simulink model "TEST_SensorSource_FromWorkspace"  (R2020b)
settings: Solver=ode1  StartTime=tspan(1)  StopTime=tspan(2)  FixedStep=1/sensorFs.imuUpdateFs  RelTol=1e-3
values from neighbouring files (symbols this model uses):
  mag1 = double([Sensors.mag1.mag_x, Sensors.mag1.mag_y, Sensors.mag1.mag_z])    [navi_marg22.m]    (also in navi_marg24.m; navi_mvo17.m)
  mag2 = double([Sensors.mag2.mag_x, Sensors.mag2.mag_y, Sensors.mag2.mag_z])    [navi_marg22.m]    (also in navi_marg24.m; navi_mvo17.m)
  time = naviRes.time    [Plot_NaviMARG.m]    (also in UAVPlotLib.m = sensors.(sensorName).time; myplot_navfilter.m = sensors.Algo.time_algo; myplot_sensor_filter_compare.m = sensors.IMU.time_imu; postplot_marg_flightdata.m = sensors.Algo.time_algo)
undefined symbols (not defined in the file or in its folder): airspeed1, airspeed2, airspeed3, baro1, IMU1, IMU1_Control, IMU2, IMU3, IN_SENSOR_SIM, laserDown1, laserDown2, radar1, radarLongDown1, radarLongForward1, ublox1, um482
settings Model: PauseTimes=266.88  Creator=sl  LastModifiedBy=sl
settings SolverCC: AutoInsertRateTranBlk=on
settings OptimizationCC: DefaultParameterBehavior=Inlined  EnhancedBackFolding=on  PassReuseOutputArgsAs=Individual arguments  ZeroExternalMemoryAtStartup=off  ZeroInternalMemoryAtStartup=off  MaxStackSize=64  OptimizeBlockOrder=speed  DifferentSizesBufferReuse=on  OptimizationCustomize=off  EfficientTunableParamExpr=on
settings DebuggingCC: MultiTaskCondExecSysMsg=none  ParameterPrecisionLossMsg=none  ParameterTunabilityLossMsg=error  UnconnectedInputMsg=none  UnconnectedOutputMsg=none  UnconnectedLineMsg=none  BusObjectLabelMismatch=error
settings HardwareCC: ProdBitPerPointer=32  ProdBitPerSizeT=32  ProdBitPerPtrDiffT=32  ProdLargestAtomicInteger=Long  ProdLargestAtomicFloat=Double  ProdWordSize=32  ProdHWDeviceType=ARM Compatible->ARM Cortex
settings ModelReferenceCC: EnableParallelModelReferenceBuilds=on  ParallelModelReferenceMATLABWorkerInit=Load Top Model
settings SFSimCC: MATLABDynamicMemAlloc=off
settings RTWCC: Description=Embedded Coder  SystemTargetFile=ert.tlc  TemplateMakefile=ert_default_tmf  GenerateReport=on  Toolchain=GNU Tools for ARM Embedded Processors  IncludeHyperlinkInReport=on  LaunchReport=on  GenerateTraceInfo=on  GenerateTraceReport=on  GenerateTraceReportSl=on  GenerateTraceReportSf=on  GenerateTraceReportEml=on
settings CodeAppCC: ForceParamTrailComments=on  IgnoreCustomStorageClasses=off  OperatorAnnotations=on  SimulinkDataObjDesc=on  SFDataObjDesc=on  InsertBlockDesc=on
settings ERTTargetCC: InlinedParameterPlacement=NonHierarchical  ERTCustomFileTemplate=example_file_process.tlc

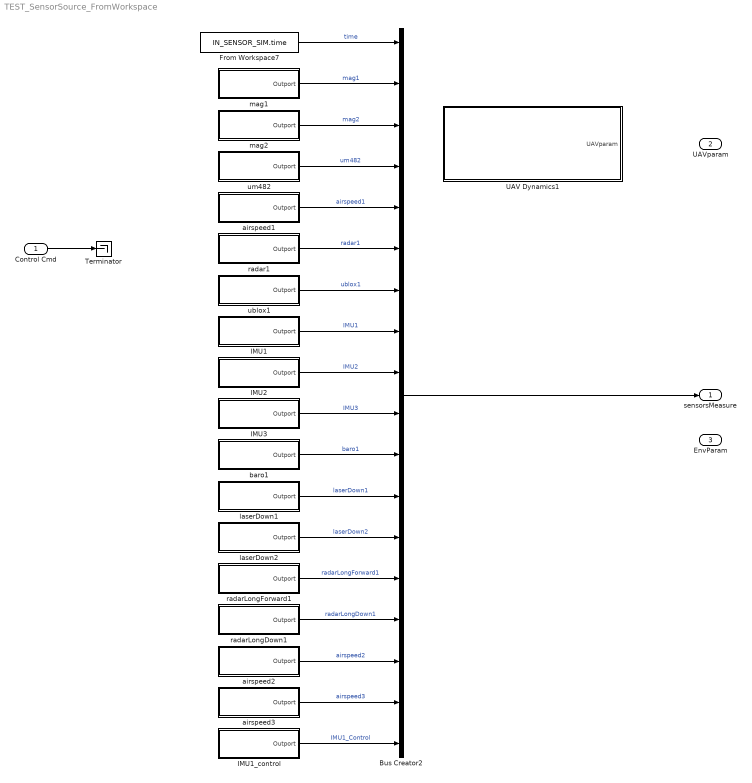
== system TEST_SensorSource_FromWorkspace ==
  Control Cmd : Inport  OutDataTypeStr=Bus: BUS_CONTROL_ACTUATOR
  Bus Creator2 : BusCreator  Inputs=time,mag1,mag2,um482,airspeed1,radar1,ublox1,IMU1,IMU2,IMU3,baro1,laserDown1,laserDown2,radarLongForward1,radarLongDown1,airspeed2,airspeed3,IMU1_Control  OutDataTypeStr=Bus: BUS_SENSOR
  From Workspace7 : FromWorkspace  VariableName=IN_SENSOR_SIM.time  OutputAfterFinalValue=Holding final value
  IMU1 : Subsystem  mask{data=IN_SENSOR_SIM.IMU1}
      mask prompts: data "IMU数据结构体"
  IMU1_control : Subsystem  mask{data=IN_SENSOR_SIM.IMU1_Control}
      mask prompts: data "IMU数据结构体"
  IMU2 : Subsystem  mask{data=IN_SENSOR_SIM.IMU2}
      mask prompts: data "IMU数据结构体"
  IMU3 : Subsystem  mask{data=IN_SENSOR_SIM.IMU3}
      mask prompts: data "IMU数据结构体"
  Terminator : Terminator
  UAV Dynamics1 : Subsystem
  airspeed1 : Subsystem  mask{data=IN_SENSOR_SIM.airspeed1}
      mask prompts: data "airspeed数据结构体"
  airspeed2 : Subsystem  mask{data=IN_SENSOR_SIM.airspeed2}
      mask prompts: data "airspeed数据结构体"
  airspeed3 : Subsystem  mask{data=IN_SENSOR_SIM.airspeed3}
      mask prompts: data "airspeed数据结构体"
  baro1 : Subsystem  mask{data=IN_SENSOR_SIM.baro1}
      mask prompts: data "baro数据结构体"
  laserDown1 : Subsystem  mask{data=IN_SENSOR_SIM.laserDown2}
      mask prompts: data "baro数据结构体"
  laserDown2 : Subsystem  mask{data=IN_SENSOR_SIM.laserDown2}
      mask prompts: data "baro数据结构体"
  mag1 : Subsystem  mask{data=IN_SENSOR_SIM.mag1}
      mask prompts: data "mag数据结构体"
  mag2 : Subsystem  mask{data=IN_SENSOR_SIM.mag2}
      mask prompts: data "mag数据结构体"
  radar1 : Subsystem  mask{data=IN_SENSOR_SIM.radar1}
      mask prompts: data "radar数据结构体"
  radarLongDown1 : Subsystem  mask{data=IN_SENSOR_SIM.radarLongDown1}
      mask prompts: data "baro数据结构体"
  radarLongForward1 : Subsystem  mask{data=IN_SENSOR_SIM.radarLongForward1}
      mask prompts: data "baro数据结构体"
  ublox1 : Subsystem  mask{data=IN_SENSOR_SIM.ublox1}
      mask prompts: data "ublox数据结构体"
  um482 : Subsystem  mask{data=IN_SENSOR_SIM.um482}
      mask prompts: data "um482数据结构体"
  sensorsMeasure : Outport  OutDataTypeStr=Bus: BUS_SENSOR
  UAVparam : Outport  Port=2  OutDataTypeStr=Bus: BUS_UAVDYN_FlightParam
  EnvParam : Outport  Port=3  OutDataTypeStr=Bus: BUS_UAVDYN_Env  LockScale=on
  wires:
  um482/1(Outport) -> Bus Creator2/4  "um482"
  Control Cmd/1 -> Terminator/1
  radarLongForward1/1(Outport) -> Bus Creator2/14  "radarLongForward1"
  radar1/1(Outport) -> Bus Creator2/6  "radar1"
  mag2/1(Outport) -> Bus Creator2/3  "mag2"
  airspeed2/1(Outport) -> Bus Creator2/16  "airspeed2"
  IMU2/1(Outport) -> Bus Creator2/9  "IMU2"
  airspeed1/1(Outport) -> Bus Creator2/5  "airspeed1"
  radarLongDown1/1(Outport) -> Bus Creator2/15  "radarLongDown1"
  From Workspace7/1 -> Bus Creator2/1  "time"
  mag1/1(Outport) -> Bus Creator2/2  "mag1"
  IMU1/1(Outport) -> Bus Creator2/8  "IMU1"
  airspeed3/1(Outport) -> Bus Creator2/17  "airspeed3"
  Bus Creator2/1 -> sensorsMeasure/1
  IMU1_control/1(Outport) -> Bus Creator2/18  "IMU1_Control"
  laserDown1/1(Outport) -> Bus Creator2/12  "laserDown1"
  baro1/1(Outport) -> Bus Creator2/11  "baro1"
  ublox1/1(Outport) -> Bus Creator2/7  "ublox1"
  laserDown2/1(Outport) -> Bus Creator2/13  "laserDown2"
  IMU3/1(Outport) -> Bus Creator2/10  "IMU3"

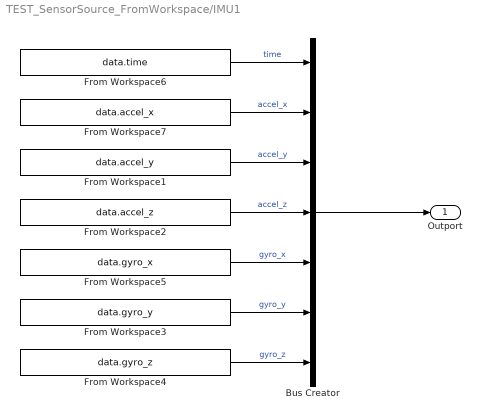
== system TEST_SensorSource_FromWorkspace/IMU1 ==
  Bus Creator : BusCreator  Inputs=7
  From Workspace1 : FromWorkspace  VariableName=data.accel_y  OutputAfterFinalValue=Holding final value
  From Workspace2 : FromWorkspace  VariableName=data.accel_z  OutputAfterFinalValue=Holding final value
  From Workspace3 : FromWorkspace  VariableName=data.gyro_y  OutputAfterFinalValue=Holding final value
  From Workspace4 : FromWorkspace  VariableName=data.gyro_z  OutputAfterFinalValue=Holding final value
  From Workspace5 : FromWorkspace  VariableName=data.gyro_x  OutputAfterFinalValue=Holding final value
  From Workspace6 : FromWorkspace  VariableName=data.time  OutputAfterFinalValue=Holding final value
  From Workspace7 : FromWorkspace  VariableName=data.accel_x  OutputAfterFinalValue=Holding final value
  Outport : Outport
  wires:
  From Workspace1/1 -> Bus Creator/3  "accel_y"
  From Workspace4/1 -> Bus Creator/7  "gyro_z"
  Bus Creator/1 -> Outport/1
  From Workspace2/1 -> Bus Creator/4  "accel_z"
  From Workspace5/1 -> Bus Creator/5  "gyro_x"
  From Workspace7/1 -> Bus Creator/2  "accel_x"
  From Workspace6/1 -> Bus Creator/1  "time"
  From Workspace3/1 -> Bus Creator/6  "gyro_y"

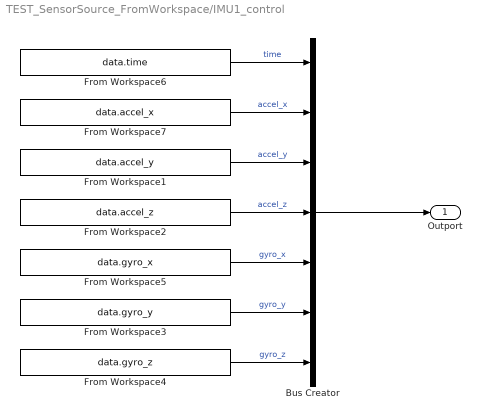
== system TEST_SensorSource_FromWorkspace/IMU1_control ==
  Bus Creator : BusCreator  Inputs=7
  From Workspace1 : FromWorkspace  VariableName=data.accel_y  OutputAfterFinalValue=Holding final value
  From Workspace2 : FromWorkspace  VariableName=data.accel_z  OutputAfterFinalValue=Holding final value
  From Workspace3 : FromWorkspace  VariableName=data.gyro_y  OutputAfterFinalValue=Holding final value
  From Workspace4 : FromWorkspace  VariableName=data.gyro_z  OutputAfterFinalValue=Holding final value
  From Workspace5 : FromWorkspace  VariableName=data.gyro_x  OutputAfterFinalValue=Holding final value
  From Workspace6 : FromWorkspace  VariableName=data.time  OutputAfterFinalValue=Holding final value
  From Workspace7 : FromWorkspace  VariableName=data.accel_x  OutputAfterFinalValue=Holding final value
  Outport : Outport
  wires:
  From Workspace3/1 -> Bus Creator/6  "gyro_y"
  From Workspace6/1 -> Bus Creator/1  "time"
  From Workspace7/1 -> Bus Creator/2  "accel_x"
  From Workspace5/1 -> Bus Creator/5  "gyro_x"
  From Workspace2/1 -> Bus Creator/4  "accel_z"
  Bus Creator/1 -> Outport/1
  From Workspace4/1 -> Bus Creator/7  "gyro_z"
  From Workspace1/1 -> Bus Creator/3  "accel_y"

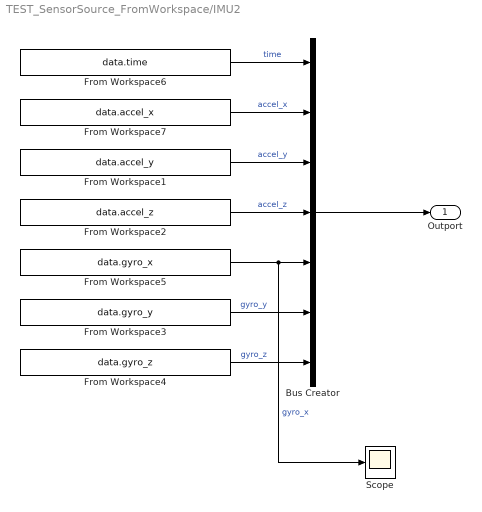
== system TEST_SensorSource_FromWorkspace/IMU2 ==
  Bus Creator : BusCreator  Inputs=7
  From Workspace1 : FromWorkspace  VariableName=data.accel_y  OutputAfterFinalValue=Holding final value
  From Workspace2 : FromWorkspace  VariableName=data.accel_z  OutputAfterFinalValue=Holding final value
  From Workspace3 : FromWorkspace  VariableName=data.gyro_y  OutputAfterFinalValue=Holding final value
  From Workspace4 : FromWorkspace  VariableName=data.gyro_z  OutputAfterFinalValue=Holding final value
  From Workspace5 : FromWorkspace  VariableName=data.gyro_x  OutputAfterFinalValue=Holding final value
  From Workspace6 : FromWorkspace  VariableName=data.time  OutputAfterFinalValue=Holding final value
  From Workspace7 : FromWorkspace  VariableName=data.accel_x  OutputAfterFinalValue=Holding final value
  Scope : Scope
  Outport : Outport
  wires:
  From Workspace3/1 -> Bus Creator/6  "gyro_y"
  From Workspace6/1 -> Bus Creator/1  "time"
  From Workspace7/1 -> Bus Creator/2  "accel_x"
  From Workspace5/1 -> Scope/1, Bus Creator/5  "gyro_x"
  From Workspace2/1 -> Bus Creator/4  "accel_z"
  Bus Creator/1 -> Outport/1
  From Workspace4/1 -> Bus Creator/7  "gyro_z"
  From Workspace1/1 -> Bus Creator/3  "accel_y"

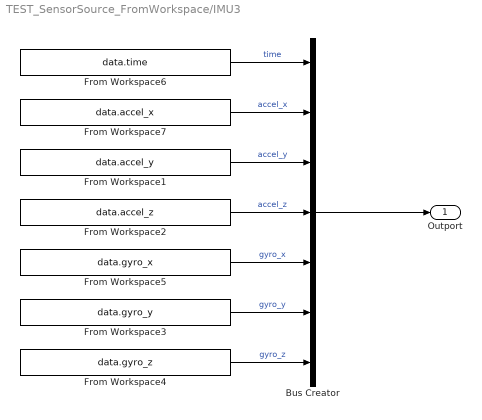
== system TEST_SensorSource_FromWorkspace/IMU3 ==
  Bus Creator : BusCreator  Inputs=7
  From Workspace1 : FromWorkspace  VariableName=data.accel_y  OutputAfterFinalValue=Holding final value
  From Workspace2 : FromWorkspace  VariableName=data.accel_z  OutputAfterFinalValue=Holding final value
  From Workspace3 : FromWorkspace  VariableName=data.gyro_y  OutputAfterFinalValue=Holding final value
  From Workspace4 : FromWorkspace  VariableName=data.gyro_z  OutputAfterFinalValue=Holding final value
  From Workspace5 : FromWorkspace  VariableName=data.gyro_x  OutputAfterFinalValue=Holding final value
  From Workspace6 : FromWorkspace  VariableName=data.time  OutputAfterFinalValue=Holding final value
  From Workspace7 : FromWorkspace  VariableName=data.accel_x  OutputAfterFinalValue=Holding final value
  Outport : Outport
  wires:
  From Workspace1/1 -> Bus Creator/3  "accel_y"
  From Workspace4/1 -> Bus Creator/7  "gyro_z"
  Bus Creator/1 -> Outport/1
  From Workspace2/1 -> Bus Creator/4  "accel_z"
  From Workspace5/1 -> Bus Creator/5  "gyro_x"
  From Workspace7/1 -> Bus Creator/2  "accel_x"
  From Workspace6/1 -> Bus Creator/1  "time"
  From Workspace3/1 -> Bus Creator/6  "gyro_y"

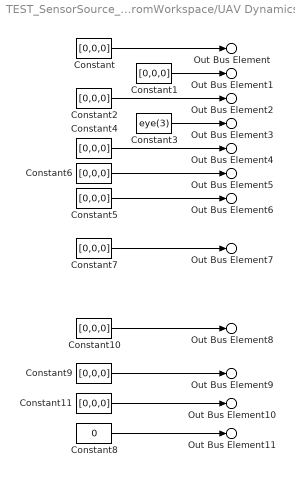
== system TEST_SensorSource_FromWorkspace/UAV Dynamics1 ==
  Constant{,1..2,4..7,9..11} (10 alike) : Constant  Value=[0,0,0]
  Constant3 : Constant  Value=eye(3)
  Constant8 : Constant  Value=0
  Out Bus Element : Outport  PortName=UAVparam  Element=vel_NED
  Out Bus Element1 : Outport  PortName=UAVparam  Element=pos_NED
  Out Bus Element2 : Outport  PortName=UAVparam  Element=euler_yaw_pitch_roll
  Out Bus Element3 : Outport  PortName=UAVparam  Element=DCMbe
  Out Bus Element4 : Outport  PortName=UAVparam  Element=vel_Body
  Out Bus Element5 : Outport  PortName=UAVparam  Element=w_Body
  Out Bus Element6 : Outport  PortName=UAVparam  Element=dw_Body
  Out Bus Element7 : Outport  PortName=UAVparam  Element=LLA
  Out Bus Element8 : Outport  PortName=UAVparam  Element=specificForce_Body
  Out Bus Element9 : Outport  PortName=UAVparam  Element=mag_Body
  Out Bus Element10 : Outport  PortName=UAVparam  Element=mag_NED
  Out Bus Element11 : Outport  PortName=UAVparam  Element=magDec_deg
  wires:
  Constant/1 -> Out Bus Element/1
  Constant1/1 -> Out Bus Element1/1
  Constant2/1 -> Out Bus Element2/1
  Constant3/1 -> Out Bus Element3/1
  Constant4/1 -> Out Bus Element4/1
  Constant6/1 -> Out Bus Element5/1
  Constant5/1 -> Out Bus Element6/1
  Constant7/1 -> Out Bus Element7/1
  Constant10/1 -> Out Bus Element8/1
  Constant9/1 -> Out Bus Element9/1
  Constant11/1 -> Out Bus Element10/1
  Constant8/1 -> Out Bus Element11/1

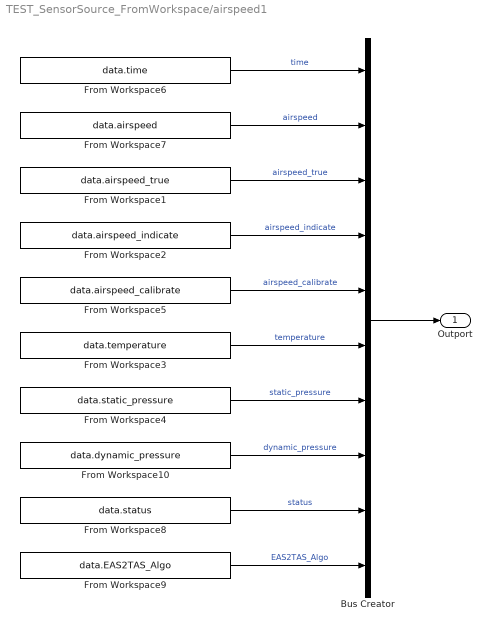
== system TEST_SensorSource_FromWorkspace/airspeed1 ==
  Bus Creator : BusCreator  Inputs=10
  From Workspace1 : FromWorkspace  VariableName=data.airspeed_true  OutputAfterFinalValue=Holding final value
  From Workspace10 : FromWorkspace  VariableName=data.dynamic_pressure  OutputAfterFinalValue=Holding final value
  From Workspace2 : FromWorkspace  VariableName=data.airspeed_indicate  OutputAfterFinalValue=Holding final value
  From Workspace3 : FromWorkspace  VariableName=data.temperature  OutputAfterFinalValue=Holding final value
  From Workspace4 : FromWorkspace  VariableName=data.static_pressure  OutputAfterFinalValue=Holding final value
  From Workspace5 : FromWorkspace  VariableName=data.airspeed_calibrate  OutputAfterFinalValue=Holding final value
  From Workspace6 : FromWorkspace  VariableName=data.time  OutputAfterFinalValue=Holding final value
  From Workspace7 : FromWorkspace  VariableName=data.airspeed  OutputAfterFinalValue=Holding final value
  From Workspace8 : FromWorkspace  VariableName=data.status  OutputAfterFinalValue=Holding final value
  From Workspace9 : FromWorkspace  VariableName=data.EAS2TAS_Algo  OutputAfterFinalValue=Holding final value
  Outport : Outport
  wires:
  Bus Creator/1 -> Outport/1
  From Workspace7/1 -> Bus Creator/2  "airspeed"
  From Workspace6/1 -> Bus Creator/1  "time"
  From Workspace1/1 -> Bus Creator/3  "airspeed_true"
  From Workspace2/1 -> Bus Creator/4  "airspeed_indicate"
  From Workspace5/1 -> Bus Creator/5  "airspeed_calibrate"
  From Workspace3/1 -> Bus Creator/6  "temperature"
  From Workspace4/1 -> Bus Creator/7  "static_pressure"
  From Workspace10/1 -> Bus Creator/8  "dynamic_pressure"
  From Workspace8/1 -> Bus Creator/9  "status"
  From Workspace9/1 -> Bus Creator/10  "EAS2TAS_Algo"

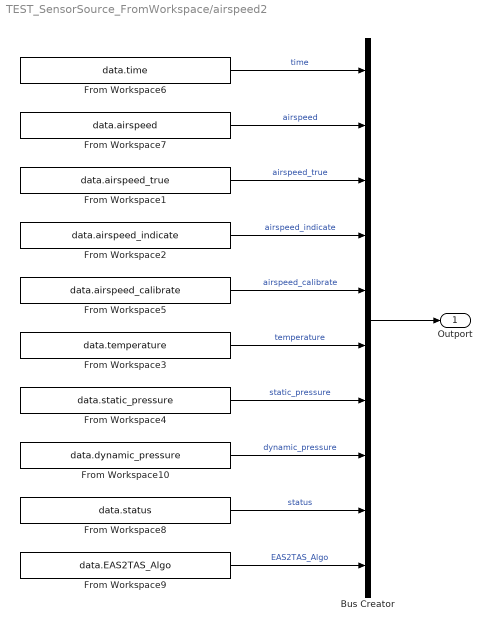
== system TEST_SensorSource_FromWorkspace/airspeed2 ==
  Bus Creator : BusCreator  Inputs=10
  From Workspace1 : FromWorkspace  VariableName=data.airspeed_true  OutputAfterFinalValue=Holding final value
  From Workspace10 : FromWorkspace  VariableName=data.dynamic_pressure  OutputAfterFinalValue=Holding final value
  From Workspace2 : FromWorkspace  VariableName=data.airspeed_indicate  OutputAfterFinalValue=Holding final value
  From Workspace3 : FromWorkspace  VariableName=data.temperature  OutputAfterFinalValue=Holding final value
  From Workspace4 : FromWorkspace  VariableName=data.static_pressure  OutputAfterFinalValue=Holding final value
  From Workspace5 : FromWorkspace  VariableName=data.airspeed_calibrate  OutputAfterFinalValue=Holding final value
  From Workspace6 : FromWorkspace  VariableName=data.time  OutputAfterFinalValue=Holding final value
  From Workspace7 : FromWorkspace  VariableName=data.airspeed  OutputAfterFinalValue=Holding final value
  From Workspace8 : FromWorkspace  VariableName=data.status  OutputAfterFinalValue=Holding final value
  From Workspace9 : FromWorkspace  VariableName=data.EAS2TAS_Algo  OutputAfterFinalValue=Holding final value
  Outport : Outport
  wires:
  From Workspace8/1 -> Bus Creator/9  "status"
  From Workspace10/1 -> Bus Creator/8  "dynamic_pressure"
  From Workspace6/1 -> Bus Creator/1  "time"
  From Workspace2/1 -> Bus Creator/4  "airspeed_indicate"
  From Workspace5/1 -> Bus Creator/5  "airspeed_calibrate"
  Bus Creator/1 -> Outport/1
  From Workspace7/1 -> Bus Creator/2  "airspeed"
  From Workspace1/1 -> Bus Creator/3  "airspeed_true"
  From Workspace4/1 -> Bus Creator/7  "static_pressure"
  From Workspace3/1 -> Bus Creator/6  "temperature"
  From Workspace9/1 -> Bus Creator/10  "EAS2TAS_Algo"

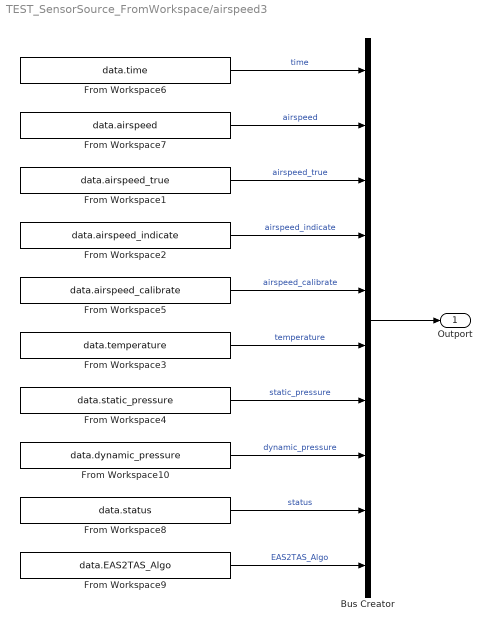
== system TEST_SensorSource_FromWorkspace/airspeed3 ==
  Bus Creator : BusCreator  Inputs=10
  From Workspace1 : FromWorkspace  VariableName=data.airspeed_true  OutputAfterFinalValue=Holding final value
  From Workspace10 : FromWorkspace  VariableName=data.dynamic_pressure  OutputAfterFinalValue=Holding final value
  From Workspace2 : FromWorkspace  VariableName=data.airspeed_indicate  OutputAfterFinalValue=Holding final value
  From Workspace3 : FromWorkspace  VariableName=data.temperature  OutputAfterFinalValue=Holding final value
  From Workspace4 : FromWorkspace  VariableName=data.static_pressure  OutputAfterFinalValue=Holding final value
  From Workspace5 : FromWorkspace  VariableName=data.airspeed_calibrate  OutputAfterFinalValue=Holding final value
  From Workspace6 : FromWorkspace  VariableName=data.time  OutputAfterFinalValue=Holding final value
  From Workspace7 : FromWorkspace  VariableName=data.airspeed  OutputAfterFinalValue=Holding final value
  From Workspace8 : FromWorkspace  VariableName=data.status  OutputAfterFinalValue=Holding final value
  From Workspace9 : FromWorkspace  VariableName=data.EAS2TAS_Algo  OutputAfterFinalValue=Holding final value
  Outport : Outport
  wires:
  From Workspace8/1 -> Bus Creator/9  "status"
  From Workspace10/1 -> Bus Creator/8  "dynamic_pressure"
  From Workspace6/1 -> Bus Creator/1  "time"
  From Workspace2/1 -> Bus Creator/4  "airspeed_indicate"
  From Workspace5/1 -> Bus Creator/5  "airspeed_calibrate"
  Bus Creator/1 -> Outport/1
  From Workspace7/1 -> Bus Creator/2  "airspeed"
  From Workspace1/1 -> Bus Creator/3  "airspeed_true"
  From Workspace4/1 -> Bus Creator/7  "static_pressure"
  From Workspace3/1 -> Bus Creator/6  "temperature"
  From Workspace9/1 -> Bus Creator/10  "EAS2TAS_Algo"

== system TEST_SensorSource_FromWorkspace/baro1 ==
  Bus Creator : BusCreator  Inputs=2
  From Workspace6 : FromWorkspace  VariableName=data.time  OutputAfterFinalValue=Holding final value
  From Workspace7 : FromWorkspace  VariableName=data.alt_baro  OutputAfterFinalValue=Holding final value
  Outport : Outport
  wires:
  From Workspace6/1 -> Bus Creator/1  "time"
  From Workspace7/1 -> Bus Creator/2  "alt_baro"
  Bus Creator/1 -> Outport/1

== system TEST_SensorSource_FromWorkspace/laserDown1 ==
  Bus Creator : BusCreator  Inputs=4
  From Workspace1 : FromWorkspace  VariableName=data.flag  OutputAfterFinalValue=Holding final value
  From Workspace2 : FromWorkspace  VariableName=data.strength  OutputAfterFinalValue=Holding final value
  From Workspace6 : FromWorkspace  VariableName=data.time  OutputAfterFinalValue=Holding final value
  From Workspace7 : FromWorkspace  VariableName=data.range  OutputAfterFinalValue=Holding final value
  Outport : Outport
  wires:
  Bus Creator/1 -> Outport/1
  From Workspace7/1 -> Bus Creator/2  "range"
  From Workspace6/1 -> Bus Creator/1  "time"
  From Workspace1/1 -> Bus Creator/3  "flag"
  From Workspace2/1 -> Bus Creator/4  "strength"

== system TEST_SensorSource_FromWorkspace/laserDown2 ==
  Bus Creator : BusCreator  Inputs=4
  From Workspace1 : FromWorkspace  VariableName=data.flag  OutputAfterFinalValue=Holding final value
  From Workspace2 : FromWorkspace  VariableName=data.strength  OutputAfterFinalValue=Holding final value
  From Workspace6 : FromWorkspace  VariableName=data.time  OutputAfterFinalValue=Holding final value
  From Workspace7 : FromWorkspace  VariableName=data.range  OutputAfterFinalValue=Holding final value
  Outport : Outport
  wires:
  From Workspace2/1 -> Bus Creator/4  "strength"
  From Workspace1/1 -> Bus Creator/3  "flag"
  From Workspace6/1 -> Bus Creator/1  "time"
  From Workspace7/1 -> Bus Creator/2  "range"
  Bus Creator/1 -> Outport/1

== system TEST_SensorSource_FromWorkspace/mag1 ==
  Bus Creator : BusCreator  Inputs=4
  From Workspace6 : FromWorkspace  VariableName=data.time  OutputAfterFinalValue=Holding final value
  mag_x : FromWorkspace  VariableName=data.mag_x  OutputAfterFinalValue=Holding final value
  mag_y : FromWorkspace  VariableName=data.mag_y  OutputAfterFinalValue=Holding final value
  mag_z : FromWorkspace  VariableName=data.mag_z  OutputAfterFinalValue=Holding final value
  Outport : Outport
  wires:
  From Workspace6/1 -> Bus Creator/1  "time"
  mag_x/1 -> Bus Creator/2  "mag_x"
  mag_z/1 -> Bus Creator/4  "mag_z"
  Bus Creator/1 -> Outport/1
  mag_y/1 -> Bus Creator/3  "mag_y"

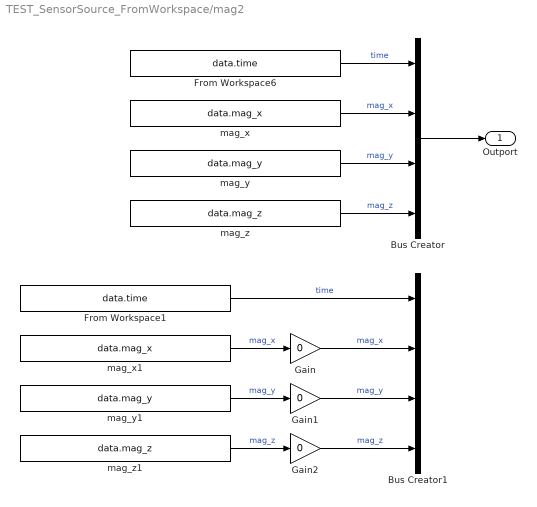
== system TEST_SensorSource_FromWorkspace/mag2 ==
  Bus Creator : BusCreator  Inputs=4
  Bus Creator1 : BusCreator  Inputs=4
  From Workspace1 : FromWorkspace  VariableName=data.time  OutputAfterFinalValue=Holding final value
  From Workspace6 : FromWorkspace  VariableName=data.time  OutputAfterFinalValue=Holding final value
  Gain : Gain  Gain=0
  Gain1 : Gain  Gain=0
  Gain2 : Gain  Gain=0
  mag_x : FromWorkspace  VariableName=data.mag_x  OutputAfterFinalValue=Holding final value
  mag_x1 : FromWorkspace  VariableName=data.mag_x  OutputAfterFinalValue=Holding final value
  mag_y : FromWorkspace  VariableName=data.mag_y  OutputAfterFinalValue=Holding final value
  mag_y1 : FromWorkspace  VariableName=data.mag_y  OutputAfterFinalValue=Holding final value
  mag_z : FromWorkspace  VariableName=data.mag_z  OutputAfterFinalValue=Holding final value
  mag_z1 : FromWorkspace  VariableName=data.mag_z  OutputAfterFinalValue=Holding final value
  Outport : Outport
  wires:
  mag_y/1 -> Bus Creator/3  "mag_y"
  mag_z/1 -> Bus Creator/4  "mag_z"
  mag_x/1 -> Bus Creator/2  "mag_x"
  From Workspace6/1 -> Bus Creator/1  "time"
  From Workspace1/1 -> Bus Creator1/1  "time"
  mag_x1/1 -> Gain/1  "mag_x"
  mag_z1/1 -> Gain2/1  "mag_z"
  mag_y1/1 -> Gain1/1  "mag_y"
  Gain/1 -> Bus Creator1/2  "mag_x"
  Gain1/1 -> Bus Creator1/3  "mag_y"
  Gain2/1 -> Bus Creator1/4  "mag_z"
  Bus Creator/1 -> Outport/1

== system TEST_SensorSource_FromWorkspace/radar1 ==
  Bus Creator : BusCreator  Inputs=4
  From Workspace1 : FromWorkspace  VariableName=data.Flag  OutputAfterFinalValue=Holding final value
  From Workspace2 : FromWorkspace  VariableName=data.Range  Interpolate=off  OutputAfterFinalValue=Holding final value
  From Workspace6 : FromWorkspace  VariableName=data.time  OutputAfterFinalValue=Holding final value
  From Workspace7 : FromWorkspace  VariableName=data.SNR  OutputAfterFinalValue=Holding final value
  Outport : Outport
  wires:
  From Workspace6/1 -> Bus Creator/1  "time"
  From Workspace7/1 -> Bus Creator/2  "SNR"
  From Workspace2/1 -> Bus Creator/4  "Range"
  Bus Creator/1 -> Outport/1
  From Workspace1/1 -> Bus Creator/3  "Flag"

== system TEST_SensorSource_FromWorkspace/radarLongDown1 ==
  Bus Creator : BusCreator  Inputs=4
  From Workspace1 : FromWorkspace  VariableName=data.flag  OutputAfterFinalValue=Holding final value
  From Workspace2 : FromWorkspace  VariableName=data.strength  OutputAfterFinalValue=Holding final value
  From Workspace6 : FromWorkspace  VariableName=data.time  OutputAfterFinalValue=Holding final value
  From Workspace7 : FromWorkspace  VariableName=data.range  OutputAfterFinalValue=Holding final value
  Outport : Outport
  wires:
  Bus Creator/1 -> Outport/1
  From Workspace7/1 -> Bus Creator/2  "range"
  From Workspace6/1 -> Bus Creator/1  "time"
  From Workspace1/1 -> Bus Creator/3  "flag"
  From Workspace2/1 -> Bus Creator/4  "strength"

== system TEST_SensorSource_FromWorkspace/radarLongForward1 ==
  Bus Creator : BusCreator  Inputs=4
  From Workspace1 : FromWorkspace  VariableName=data.flag  OutputAfterFinalValue=Holding final value
  From Workspace2 : FromWorkspace  VariableName=data.strength  OutputAfterFinalValue=Holding final value
  From Workspace6 : FromWorkspace  VariableName=data.time  OutputAfterFinalValue=Holding final value
  From Workspace7 : FromWorkspace  VariableName=data.range  OutputAfterFinalValue=Holding final value
  Outport : Outport
  wires:
  From Workspace2/1 -> Bus Creator/4  "strength"
  From Workspace1/1 -> Bus Creator/3  "flag"
  From Workspace6/1 -> Bus Creator/1  "time"
  From Workspace7/1 -> Bus Creator/2  "range"
  Bus Creator/1 -> Outport/1

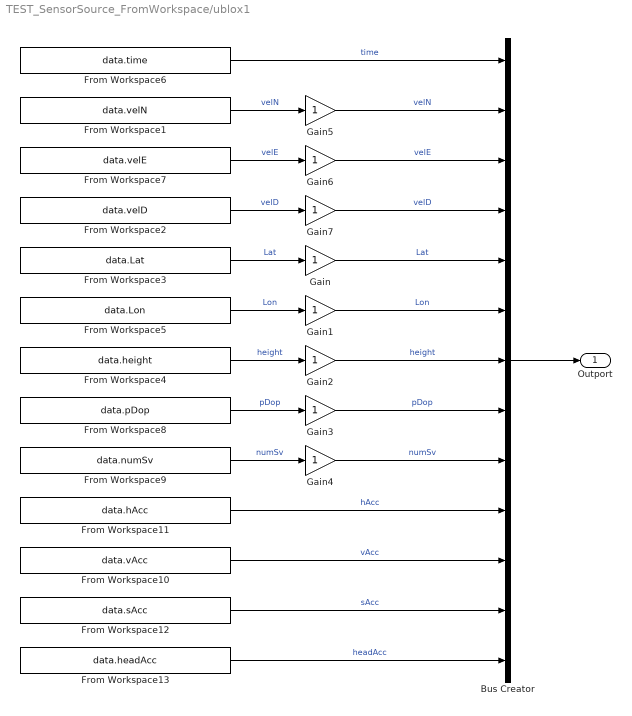
== system TEST_SensorSource_FromWorkspace/ublox1 ==
  Bus Creator : BusCreator  Inputs=13
  From Workspace1 : FromWorkspace  VariableName=data.velN  OutputAfterFinalValue=Holding final value
  From Workspace10 : FromWorkspace  VariableName=data.vAcc  OutputAfterFinalValue=Holding final value
  From Workspace11 : FromWorkspace  VariableName=data.hAcc  OutputAfterFinalValue=Holding final value
  From Workspace12 : FromWorkspace  VariableName=data.sAcc  OutputAfterFinalValue=Holding final value
  From Workspace13 : FromWorkspace  VariableName=data.headAcc  OutputAfterFinalValue=Holding final value
  From Workspace2 : FromWorkspace  VariableName=data.velD  OutputAfterFinalValue=Holding final value
  From Workspace3 : FromWorkspace  VariableName=data.Lat  OutputAfterFinalValue=Holding final value
  From Workspace4 : FromWorkspace  VariableName=data.height  OutputAfterFinalValue=Holding final value
  From Workspace5 : FromWorkspace  VariableName=data.Lon  OutputAfterFinalValue=Holding final value
  From Workspace6 : FromWorkspace  VariableName=data.time  OutputAfterFinalValue=Holding final value
  From Workspace7 : FromWorkspace  VariableName=data.velE  OutputAfterFinalValue=Holding final value
  From Workspace8 : FromWorkspace  VariableName=data.pDop  OutputAfterFinalValue=Holding final value
  From Workspace9 : FromWorkspace  VariableName=data.numSv  OutputAfterFinalValue=Holding final value
  Gain{,1..7} (8 alike) : Gain
  Outport : Outport
  wires:
  From Workspace9/1 -> Gain4/1  "numSv"
  From Workspace8/1 -> Gain3/1  "pDop"
  From Workspace4/1 -> Gain2/1  "height"
  Bus Creator/1 -> Outport/1
  From Workspace3/1 -> Gain/1  "Lat"
  From Workspace6/1 -> Bus Creator/1  "time"
  From Workspace5/1 -> Gain1/1  "Lon"
  From Workspace1/1 -> Gain5/1  "velN"
  From Workspace7/1 -> Gain6/1  "velE"
  From Workspace2/1 -> Gain7/1  "velD"
  From Workspace11/1 -> Bus Creator/10  "hAcc"
  From Workspace10/1 -> Bus Creator/11  "vAcc"
  From Workspace12/1 -> Bus Creator/12  "sAcc"
  From Workspace13/1 -> Bus Creator/13  "headAcc"
  Gain/1 -> Bus Creator/5  "Lat"
  Gain1/1 -> Bus Creator/6  "Lon"
  Gain2/1 -> Bus Creator/7  "height"
  Gain3/1 -> Bus Creator/8  "pDop"
  Gain4/1 -> Bus Creator/9  "numSv"
  Gain5/1 -> Bus Creator/2  "velN"
  Gain6/1 -> Bus Creator/3  "velE"
  Gain7/1 -> Bus Creator/4  "velD"

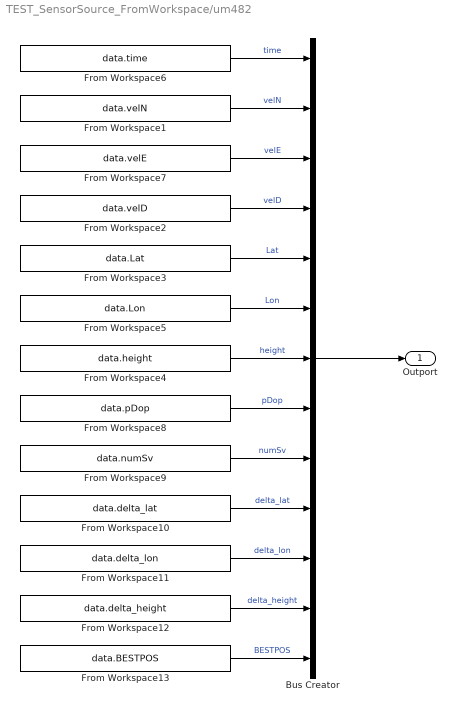
== system TEST_SensorSource_FromWorkspace/um482 ==
  Bus Creator : BusCreator  Inputs=13
  From Workspace1 : FromWorkspace  VariableName=data.velN  OutputAfterFinalValue=Holding final value
  From Workspace10 : FromWorkspace  VariableName=data.delta_lat  OutputAfterFinalValue=Holding final value
  From Workspace11 : FromWorkspace  VariableName=data.delta_lon  OutputAfterFinalValue=Holding final value
  From Workspace12 : FromWorkspace  VariableName=data.delta_height  OutputAfterFinalValue=Holding final value
  From Workspace13 : FromWorkspace  VariableName=data.BESTPOS  OutputAfterFinalValue=Holding final value
  From Workspace2 : FromWorkspace  VariableName=data.velD  OutputAfterFinalValue=Holding final value
  From Workspace3 : FromWorkspace  VariableName=data.Lat  OutputAfterFinalValue=Holding final value
  From Workspace4 : FromWorkspace  VariableName=data.height  OutputAfterFinalValue=Holding final value
  From Workspace5 : FromWorkspace  VariableName=data.Lon  OutputAfterFinalValue=Holding final value
  From Workspace6 : FromWorkspace  VariableName=data.time  OutputAfterFinalValue=Holding final value
  From Workspace7 : FromWorkspace  VariableName=data.velE  OutputAfterFinalValue=Holding final value
  From Workspace8 : FromWorkspace  VariableName=data.pDop  OutputAfterFinalValue=Holding final value
  From Workspace9 : FromWorkspace  VariableName=data.numSv  OutputAfterFinalValue=Holding final value
  Outport : Outport
  wires:
  Bus Creator/1 -> Outport/1
  From Workspace3/1 -> Bus Creator/5  "Lat"
  From Workspace4/1 -> Bus Creator/7  "height"
  From Workspace7/1 -> Bus Creator/3  "velE"
  From Workspace9/1 -> Bus Creator/9  "numSv"
  From Workspace2/1 -> Bus Creator/4  "velD"
  From Workspace6/1 -> Bus Creator/1  "time"
  From Workspace1/1 -> Bus Creator/2  "velN"
  From Workspace5/1 -> Bus Creator/6  "Lon"
  From Workspace8/1 -> Bus Creator/8  "pDop"
  From Workspace10/1 -> Bus Creator/10  "delta_lat"
  From Workspace11/1 -> Bus Creator/11  "delta_lon"
  From Workspace12/1 -> Bus Creator/12  "delta_height"
  From Workspace13/1 -> Bus Creator/13  "BESTPOS"
